simulink model "Kinematics_switch_sim"  (R2023b)
settings: Solver=ode15s  StartTime=0.0  StopTime=60  FixedStep=0.01  MaxStep=0.1  RelTol=1e-5
values from neighbouring files (symbols this model uses):
  a = 6.851221970532768e3    (= 6851.22197053)    [Kinematics_switch.m]
  A_313 = ( R_om * R_i * R_OM ).'    [Kinematics_switch.m]
  e = 0.001830122216180    (= 0.00183012221618)    [Kinematics_switch.m]
  I = diag([Ix Iy Iz])    [Kinematics_switch.m]
  I_inv = inv(I)    [Kinematics_switch.m]
  n = sqrt(mu / a^3)    [Kinematics_switch.m]
  s0 = [0; asin(0.4); pi/3]    [Kinematics_switch.m]
  theta0 = 3.109851878856139    (= 3.10985187886)    [Kinematics_switch.m]
  tol = 0.2    [Kinematics_switch.m]
  w0 = [0.5; -0.2; 1.0]    [Kinematics_switch.m]
libraries: simulink x2, matrix_library x1
settings Model: PauseTimes=53.05  Creator=turcu  LastModifiedBy=turcu

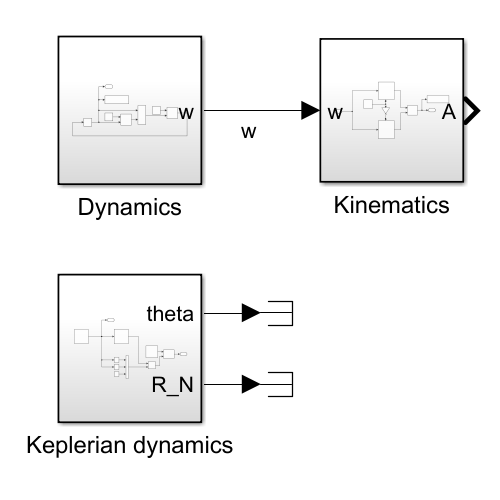
[thumbnail: Simulink's stored preview of the top-level diagram]
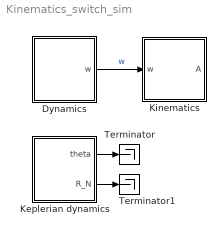
== system Kinematics_switch_sim ==
  Dynamics : Subsystem
  Keplerian dynamics : Subsystem
  Kinematics : Subsystem
  Terminator : Terminator
  Terminator1 : Terminator
  wires:
  Dynamics/1(w) -> Kinematics/1(w)  "w"
  Keplerian dynamics/1(theta) -> Terminator/1
  Keplerian dynamics/2(R_N) -> Terminator1/1

== system Kinematics_switch_sim/Dynamics ==
  Constant : Constant  Value=I
  Constant1 : Constant  Value=-I_inv
  Cross Product : matrix_library/Cross Product
  Integrator : Integrator  InitialCondition=w0
  Product : Product  Multiplication=Matrix(*)
  Product1 : Product  Multiplication=Matrix(*)
  To Workspace : ToWorkspace  VariableName=w  SaveFormat=Timeseries  SampleTime=-1
  w : Outport
  wires:
  Cross Product/1 -> Product1/2
  Constant/1 -> Product/1
  Integrator/1 -> Product/2, w/1, To Workspace/1, Cross Product/1  "w"
  Constant1/1 -> Product1/1
  Product/1 -> Cross Product/2
  Product1/1 -> Integrator/1  "wdot"

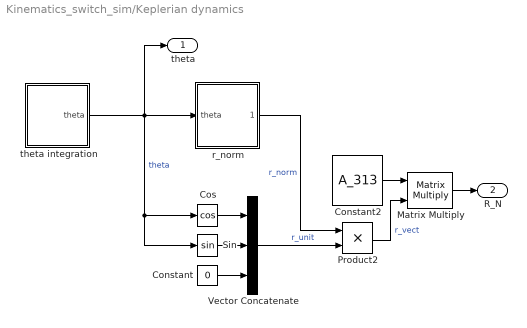
== system Kinematics_switch_sim/Keplerian dynamics ==
  Constant : Constant  Value=0
  Constant2 : Constant  Value=A_313
  Cos : Trigonometry  Operator=cos
  Matrix Multiply : Product  Multiplication=Matrix(*)
  Product2 : Product
  Sin : Trigonometry
  Vector Concatenate : Concatenate  NumInputs=3
  r_norm : Subsystem
  theta integration : Subsystem
  theta : Outport
  R_N : Outport  Port=2
  wires:
  Constant/1 -> Vector Concatenate/3
  Cos/1 -> Vector Concatenate/1
  r_norm/1(r_norm) -> Product2/1  "r_norm"
  Vector Concatenate/1 -> Product2/2  "r_unit"
  Sin/1 -> Vector Concatenate/2
  Constant2/1 -> Matrix Multiply/1
  Product2/1 -> Matrix Multiply/2  "r_vect"
  Matrix Multiply/1 -> R_N/1
  theta integration/1(theta) -> theta/1, Sin/1, Cos/1, r_norm/1(theta)  "theta"

== system Kinematics_switch_sim/Kinematics ==
  w : Inport
  Kinematics 312 : Subsystem
  Kinematics 313 : Subsystem
  Merge : Merge
  NOT : Logic  Operator=NOT  IconShape=distinctive  AllPortsSameDT=off  OutDataTypeStr=boolean
  System switcher : Subsystem
  To Workspace : ToWorkspace  VariableName=A  SaveFormat=Timeseries  SampleTime=-1
  A : Outport
  wires:
  NOT/1 -> Kinematics 313/Enable
  w/1 -> Kinematics 312/1(w), Kinematics 313/1(w)
  System switcher/1(flag) -> Kinematics 312/Enable, NOT/1
  Kinematics 313/1(A) -> Merge/2
  Merge/1 -> A/1, To Workspace/1  "A"
  Kinematics 312/1(A) -> Merge/1

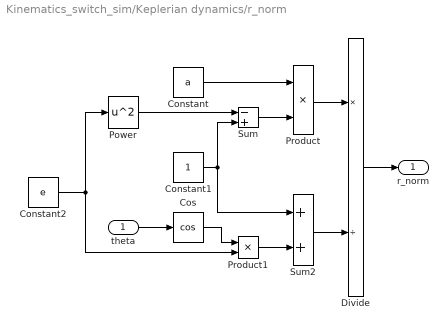
== system Kinematics_switch_sim/Keplerian dynamics/r_norm ==
  theta : Inport
  Constant : Constant  Value=a
  Constant1 : Constant
  Constant2 : Constant  Value=e
  Cos : Trigonometry  Operator=cos
  Divide : Product  Inputs=*/
  Power : Math  Operator=square
  Product : Product
  Product1 : Product
  Sum : Sum  Inputs=-+
  Sum2 : Sum
  r_norm : Outport
  wires:
  Constant2/1 -> Product1/2, Power/1
  Constant1/1 -> Sum/2, Sum2/1
  Sum/1 -> Product/2
  Constant/1 -> Product/1
  theta/1 -> Cos/1
  Cos/1 -> Product1/1
  Divide/1 -> r_norm/1
  Sum2/1 -> Divide/2
  Product/1 -> Divide/1
  Product1/1 -> Sum2/2
  Power/1 -> Sum/1

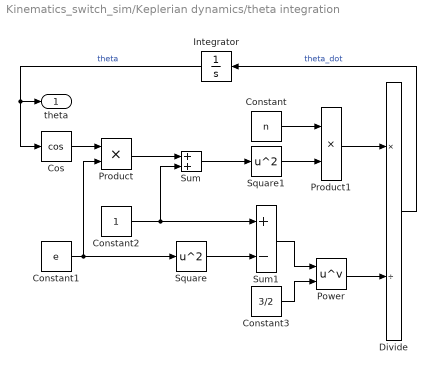
== system Kinematics_switch_sim/Keplerian dynamics/theta integration ==
  Constant : Constant  Value=n
  Constant1 : Constant  Value=e
  Constant2 : Constant
  Constant3 : Constant  Value=3/2
  Cos : Trigonometry  Operator=cos
  Divide : Product  Inputs=*/
  Integrator : Integrator  InitialCondition=theta0
  Power : Math  Operator=pow
  Product : Product
  Product1 : Product
  Square : Math  Operator=square
  Square1 : Math  Operator=square
  Sum : Sum
  Sum1 : Sum  Inputs=+-
  theta : Outport
  wires:
  Product1/1 -> Divide/1
  Power/1 -> Divide/2
  Sum1/1 -> Power/1
  Constant2/1 -> Sum/2, Sum1/1
  Square/1 -> Sum1/2
  Constant1/1 -> Product/2, Square/1
  Constant/1 -> Product1/1
  Sum/1 -> Square1/1
  Square1/1 -> Product1/2
  Cos/1 -> Product/1
  Divide/1 -> Integrator/1  "theta_dot"
  Integrator/1 -> theta/1, Cos/1  "theta"
  Constant3/1 -> Power/2
  Product/1 -> Sum/1

== system Kinematics_switch_sim/Kinematics/Kinematics 312 ==
  w : Inport
  Enable : EnablePort  StatesWhenEnabling=reset
  A - s_312 : Subsystem
  Euler angles : Subsystem
  IC : InitialCondition  Value=s0
  s_312 - A : Subsystem
  s_313 - A : Subsystem
  A : Outport
  wires:
  s_312 - A/1(A) -> A/1  "A"
  Euler angles/1(s) -> s_312 - A/1(s)  "s"
  w/1 -> Euler angles/1(w)
  IC/1 -> Euler angles/2(s0)
  A - s_312/1(s) -> IC/1
  s_313 - A/1(A) -> A - s_312/1(A)
  [s_313] -> s_313 - A/1(s)

== system Kinematics_switch_sim/Kinematics/Kinematics 313 ==
  w : Inport
  Enable : EnablePort  StatesWhenEnabling=reset
  A - s_313 : Subsystem
  Euler angles : Subsystem
  s_312 - A : Subsystem
  s_313 - A : Subsystem
  A : Outport
  wires:
  w/1 -> Euler angles/1(w)
  Euler angles/1(s) -> s_313 - A/1(s)
  s_313 - A/1(A) -> A/1
  A - s_313/1(s) -> Euler angles/2(s0)
  s_312 - A/1(A) -> A - s_313/1(A)
  [s_312] -> s_312 - A/1(s)

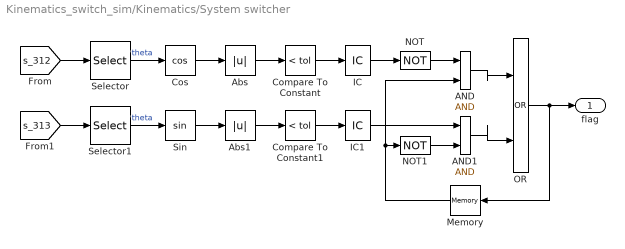
== system Kinematics_switch_sim/Kinematics/System switcher ==
  AND : Logic  IconShape=distinctive  AllPortsSameDT=off  OutDataTypeStr=boolean
  AND1 : Logic  IconShape=distinctive  AllPortsSameDT=off  OutDataTypeStr=boolean
  Abs : Abs  SaturateOnIntegerOverflow=off
  Abs1 : Abs  SaturateOnIntegerOverflow=off
  Compare To Constant : simulink/Logic and Bit Operations/Compare To Constant  relop=<  const=tol  OutDataTypeStr=boolean
  Compare To Constant1 : simulink/Logic and Bit Operations/Compare To Constant  relop=<  const=tol  OutDataTypeStr=boolean
  Cos : Trigonometry  Operator=cos
  IC : InitialCondition  Value=0
  IC1 : InitialCondition  Value=0
  Memory : Memory  InitialCondition=1
  NOT : Logic  Operator=NOT  IconShape=distinctive  AllPortsSameDT=off  OutDataTypeStr=boolean
  NOT1 : Logic  Operator=NOT  IconShape=distinctive  AllPortsSameDT=off  OutDataTypeStr=boolean
  OR : Logic  Operator=OR  IconShape=distinctive  AllPortsSameDT=off  OutDataTypeStr=boolean
  Selector : Selector  InputPortWidth=3  IndexOptions=Index vector (dialog)  Indices=2  OutputSizes=1
  Selector1 : Selector  InputPortWidth=3  IndexOptions=Index vector (dialog)  Indices=2  OutputSizes=1
  Sin : Trigonometry
  flag : Outport
  wires:
  Cos/1 -> Abs/1
  [s_312] -> Selector/1
  Compare To Constant/1 -> IC/1
  Selector1/1 -> Sin/1  "theta"
  Abs/1 -> Compare To Constant/1
  Compare To Constant1/1 -> IC1/1
  Selector/1 -> Cos/1  "theta"
  Abs1/1 -> Compare To Constant1/1
  Sin/1 -> Abs1/1
  [s_313] -> Selector1/1
  IC/1 -> NOT/1
  NOT/1 -> AND/1
  AND/1 -> OR/1
  NOT1/1 -> AND1/2
  IC1/1 -> AND1/1
  AND1/1 -> OR/2
  OR/1 -> Memory/1, flag/1
  Memory/1 -> AND/2, NOT1/1

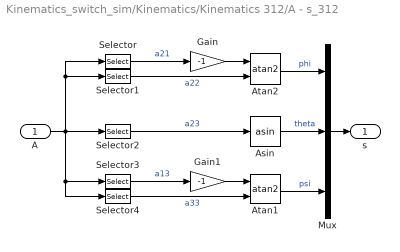
== system Kinematics_switch_sim/Kinematics/Kinematics 312/A - s_312 ==
  A : Inport
  Asin : Trigonometry  Operator=asin
  Atan1 : Trigonometry  Operator=atan2
  Atan2 : Trigonometry  Operator=atan2
  Gain : Gain  Gain=-1
  Gain1 : Gain  Gain=-1
  Mux : Mux  Inputs=3
  Selector : Selector  NumberOfDimensions=2  InputPortWidth=3  IndexOptions=Index vector (dialog),Index vector (dialog)  Indices=2,1  OutputSizes=1,1
  Selector1 : Selector  NumberOfDimensions=2  InputPortWidth=3  IndexOptions=Index vector (dialog),Index vector (dialog)  Indices=2,2  OutputSizes=1,1
  Selector2 : Selector  NumberOfDimensions=2  InputPortWidth=3  IndexOptions=Index vector (dialog),Index vector (dialog)  Indices=2,3  OutputSizes=1,1
  Selector3 : Selector  NumberOfDimensions=2  InputPortWidth=3  IndexOptions=Index vector (dialog),Index vector (dialog)  Indices=1,3  OutputSizes=1,1
  Selector4 : Selector  NumberOfDimensions=2  InputPortWidth=3  IndexOptions=Index vector (dialog),Index vector (dialog)  Indices=3,3  OutputSizes=1,1
  s : Outport
  wires:
  Mux/1 -> s/1
  Selector4/1 -> Atan1/2  "a33"
  Atan1/1 -> Mux/3  "psi"
  Atan2/1 -> Mux/1  "phi"
  A/1 -> Selector2/1, Selector1/1, Selector/1, Selector3/1, Selector4/1
  Selector2/1 -> Asin/1  "a23"
  Selector3/1 -> Gain1/1  "a13"
  Selector1/1 -> Atan2/2  "a22"
  Selector/1 -> Gain/1  "a21"
  Asin/1 -> Mux/2  "theta"
  Gain/1 -> Atan2/1
  Gain1/1 -> Atan1/1

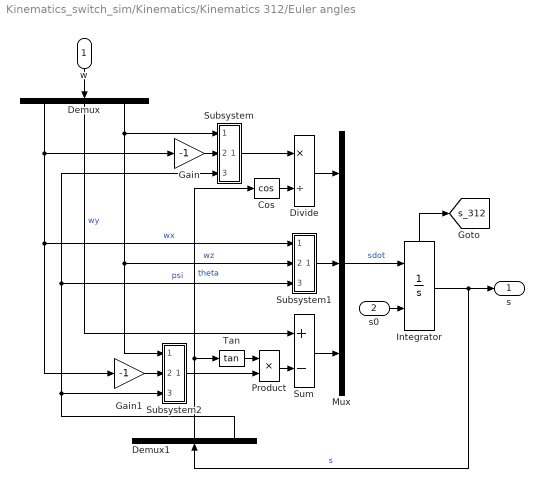
== system Kinematics_switch_sim/Kinematics/Kinematics 312/Euler angles ==
  w : Inport
  s0 : Inport  Port=2
  Cos : Trigonometry  Operator=cos
  Demux : Demux  Outputs=3
  Demux1 : Demux  Outputs=3
  Divide : Product  Inputs=*/
  Gain : Gain  Gain=-1
  Gain1 : Gain  Gain=-1
  Integrator : Integrator  InitialConditionSource=external  InitialCondition=s0  WrapState=on  WrappedStateUpperValue=2*pi  WrappedStateLowerValue=0  ShowStatePort=on
  Mux : Mux  Inputs=3
  Product : Product
  Subsystem : Subsystem
  Subsystem1 : Subsystem
  Subsystem2 : Subsystem
  Sum : Sum  Inputs=+-
  Tan : Trigonometry  Operator=tan
  s : Outport
  tag scope: s_312=global
  wires:
  w/1 -> Demux/1
  Integrator/1 -> Demux1/1, s/1  "s"
  Demux/3 -> Subsystem2/1(In1), Subsystem1/2(In2), Subsystem/1(In1)  "wz"
  Gain/1 -> Subsystem/2(In2)
  Demux/1 -> Gain1/1, Subsystem1/1(In1), Gain/1  "wx"
  Demux1/3 -> Subsystem2/3(In3), Subsystem1/3(In3), Subsystem/3(In3)  "psi"
  Subsystem/1(Out1) -> Divide/1
  Cos/1 -> Divide/2
  Demux1/2 -> Cos/1, Tan/1  "theta"
  Divide/1 -> Mux/1
  Subsystem1/1(Out1) -> Mux/2
  Gain1/1 -> Subsystem2/2(In2)
  Tan/1 -> Product/1
  Subsystem2/1(Out1) -> Product/2
  Product/1 -> Sum/2
  Demux/2 -> Sum/1  "wy"
  Sum/1 -> Mux/3
  Mux/1 -> Integrator/1  "sdot"
  s0/1 -> Integrator/2
  Integrator/State -> [s_312]

== system Kinematics_switch_sim/Kinematics/Kinematics 312/s_312 - A ==
  s : Inport
  Demux : Demux  Outputs=3
  Product : Product  Inputs=3  Multiplication=Matrix(*)
  R1 : Subsystem
  R2 : Subsystem
  R3 : Subsystem
  A : Outport
  wires:
  s/1 -> Demux/1  "s"
  R1/1(R1) -> Product/2
  R3/1(R3) -> Product/3
  R2/1(R2) -> Product/1
  Product/1 -> A/1
  Demux/2 -> R1/1(x)  "theta"
  Demux/1 -> R3/1(x)  "phi"
  Demux/3 -> R2/1(x)  "psi"

== system Kinematics_switch_sim/Kinematics/Kinematics 312/s_313 - A ==
  s : Inport
  Demux : Demux  Outputs=3
  Product : Product  Inputs=3  Multiplication=Matrix(*)
  R1 : Subsystem
  R3_1 : Subsystem
  R3_2 : Subsystem
  A : Outport
  wires:
  Demux/3 -> R3_2/1(x)  "psi"
  Demux/1 -> R3_1/1(x)  "phi"
  Demux/2 -> R1/1(x)  "theta"
  Product/1 -> A/1
  R1/1(R1) -> Product/2
  s/1 -> Demux/1  "s"
  R3_1/1(R3) -> Product/3
  R3_2/1(R3) -> Product/1

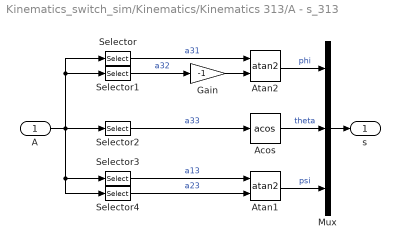
== system Kinematics_switch_sim/Kinematics/Kinematics 313/A - s_313 ==
  A : Inport
  Acos : Trigonometry  Operator=acos
  Atan1 : Trigonometry  Operator=atan2
  Atan2 : Trigonometry  Operator=atan2
  Gain : Gain  Gain=-1
  Mux : Mux  Inputs=3
  Selector : Selector  NumberOfDimensions=2  InputPortWidth=3  IndexOptions=Index vector (dialog),Index vector (dialog)  Indices=3,1  OutputSizes=1,1
  Selector1 : Selector  NumberOfDimensions=2  InputPortWidth=3  IndexOptions=Index vector (dialog),Index vector (dialog)  Indices=3,2  OutputSizes=1,1
  Selector2 : Selector  NumberOfDimensions=2  InputPortWidth=3  IndexOptions=Index vector (dialog),Index vector (dialog)  Indices=3,3  OutputSizes=1,1
  Selector3 : Selector  NumberOfDimensions=2  InputPortWidth=3  IndexOptions=Index vector (dialog),Index vector (dialog)  Indices=1,3  OutputSizes=1,1
  Selector4 : Selector  NumberOfDimensions=2  InputPortWidth=3  IndexOptions=Index vector (dialog),Index vector (dialog)  Indices=2,3  OutputSizes=1,1
  s : Outport
  wires:
  Acos/1 -> Mux/2  "theta"
  Selector/1 -> Atan2/1  "a31"
  Selector1/1 -> Gain/1  "a32"
  Selector3/1 -> Atan1/1  "a13"
  Selector2/1 -> Acos/1  "a33"
  A/1 -> Selector4/1, Selector3/1, Selector/1, Selector1/1, Selector2/1
  Atan2/1 -> Mux/1  "phi"
  Atan1/1 -> Mux/3  "psi"
  Gain/1 -> Atan2/2
  Selector4/1 -> Atan1/2  "a23"
  Mux/1 -> s/1

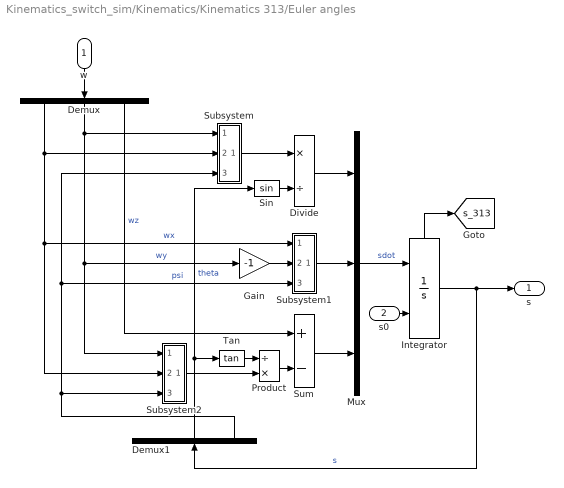
== system Kinematics_switch_sim/Kinematics/Kinematics 313/Euler angles ==
  w : Inport
  s0 : Inport  Port=2
  Demux : Demux  Outputs=3
  Demux1 : Demux  Outputs=3
  Divide : Product  Inputs=*/
  Gain : Gain  Gain=-1
  Integrator : Integrator  InitialConditionSource=external  InitialCondition=s0  WrapState=on  WrappedStateUpperValue=2*pi  WrappedStateLowerValue=0  ShowStatePort=on
  Mux : Mux  Inputs=3
  Product : Product  Inputs=/*
  Sin : Trigonometry
  Subsystem : Subsystem
  Subsystem1 : Subsystem
  Subsystem2 : Subsystem
  Sum : Sum  Inputs=+-
  Tan : Trigonometry  Operator=tan
  s : Outport
  tag scope: s_313=global
  wires:
  Mux/1 -> Integrator/1  "sdot"
  Sum/1 -> Mux/3
  Demux/2 -> Subsystem/1(In1), Subsystem2/1(In1), Gain/1  "wy"
  Product/1 -> Sum/2
  Subsystem2/1(Out1) -> Product/2
  Tan/1 -> Product/1
  Subsystem1/1(Out1) -> Mux/2
  Divide/1 -> Mux/1
  Demux1/2 -> Sin/1, Tan/1  "theta"
  Subsystem/1(Out1) -> Divide/1
  Demux1/3 -> Subsystem/3(In3), Subsystem1/3(In3), Subsystem2/3(In3)  "psi"
  Demux/1 -> Subsystem2/2(In2), Subsystem1/1(In1), Subsystem/2(In2)  "wx"
  Demux/3 -> Sum/1  "wz"
  Integrator/1 -> Demux1/1, s/1  "s"
  w/1 -> Demux/1
  Sin/1 -> Divide/2
  Gain/1 -> Subsystem1/2(In2)
  s0/1 -> Integrator/2
  Integrator/State -> [s_313]

== system Kinematics_switch_sim/Kinematics/Kinematics 313/s_312 - A ==
  s : Inport
  Demux : Demux  Outputs=3
  Product : Product  Inputs=3  Multiplication=Matrix(*)
  R1 : Subsystem
  R2 : Subsystem
  R3 : Subsystem
  A : Outport
  wires:
  s/1 -> Demux/1  "s"
  R1/1(R1) -> Product/2
  R3/1(R3) -> Product/3
  R2/1(R2) -> Product/1
  Product/1 -> A/1
  Demux/2 -> R1/1(x)  "theta"
  Demux/1 -> R3/1(x)  "phi"
  Demux/3 -> R2/1(x)  "psi"

== system Kinematics_switch_sim/Kinematics/Kinematics 313/s_313 - A ==
  s : Inport
  Demux : Demux  Outputs=3
  Product : Product  Inputs=3  Multiplication=Matrix(*)
  R1 : Subsystem
  R3_1 : Subsystem
  R3_2 : Subsystem
  A : Outport
  wires:
  Demux/3 -> R3_2/1(x)  "psi"
  Demux/1 -> R3_1/1(x)  "phi"
  Demux/2 -> R1/1(x)  "theta"
  Product/1 -> A/1
  R1/1(R1) -> Product/2
  s/1 -> Demux/1  "s"
  R3_1/1(R3) -> Product/3
  R3_2/1(R3) -> Product/1

== system Kinematics_switch_sim/Kinematics/Kinematics 312/Euler angles/Subsystem ==
  In1 : Inport
  In2 : Inport  Port=2
  In3 : Inport  Port=3
  Cos : Trigonometry  Operator=cos
  Product : Product
  Product1 : Product
  Sin : Trigonometry
  Sum : Sum
  Out1 : Outport
  wires:
  In3/1 -> Sin/1, Cos/1
  In1/1 -> Product/1
  Cos/1 -> Product/2
  Sin/1 -> Product1/1
  In2/1 -> Product1/2
  Product/1 -> Sum/1
  Product1/1 -> Sum/2
  Sum/1 -> Out1/1

== system Kinematics_switch_sim/Kinematics/Kinematics 312/Euler angles/Subsystem1 ==
  In1 : Inport
  In2 : Inport  Port=2
  In3 : Inport  Port=3
  Cos : Trigonometry  Operator=cos
  Product : Product
  Product1 : Product
  Sin : Trigonometry
  Sum : Sum
  Out1 : Outport
  wires:
  Sum/1 -> Out1/1
  Product1/1 -> Sum/2
  Product/1 -> Sum/1
  In2/1 -> Product1/2
  Sin/1 -> Product1/1
  Cos/1 -> Product/2
  In1/1 -> Product/1
  In3/1 -> Cos/1, Sin/1

== system Kinematics_switch_sim/Kinematics/Kinematics 312/Euler angles/Subsystem2 ==
  In1 : Inport
  In2 : Inport  Port=2
  In3 : Inport  Port=3
  Cos : Trigonometry  Operator=cos
  Product : Product
  Product1 : Product
  Sin : Trigonometry
  Sum : Sum
  Out1 : Outport
  wires:
  In3/1 -> Sin/1, Cos/1
  In1/1 -> Product/1
  Cos/1 -> Product/2
  Sin/1 -> Product1/1
  In2/1 -> Product1/2
  Product/1 -> Sum/1
  Product1/1 -> Sum/2
  Sum/1 -> Out1/1

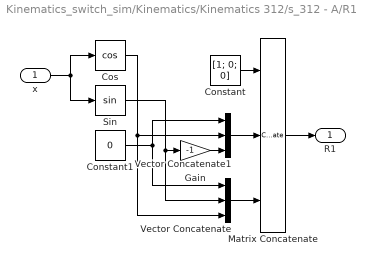
== system Kinematics_switch_sim/Kinematics/Kinematics 312/s_312 - A/R1 ==
  x : Inport
  Constant : Constant  Value=[1; 0; 0]
  Constant1 : Constant  Value=0
  Cos : Trigonometry  Operator=cos
  Gain : Gain  Gain=-1
  Matrix Concatenate : Concatenate  NumInputs=3  Mode=Multidimensional array  ConcatenateDimension=2
  Sin : Trigonometry
  Vector Concatenate : Concatenate  NumInputs=3
  Vector Concatenate1 : Concatenate  NumInputs=3
  R1 : Outport
  wires:
  Matrix Concatenate/1 -> R1/1
  x/1 -> Cos/1, Sin/1
  Vector Concatenate1/1 -> Matrix Concatenate/2
  Constant/1 -> Matrix Concatenate/1
  Vector Concatenate/1 -> Matrix Concatenate/3
  Constant1/1 -> Vector Concatenate/1, Vector Concatenate1/1
  Cos/1 -> Vector Concatenate/3, Vector Concatenate1/2
  Gain/1 -> Vector Concatenate1/3
  Sin/1 -> Vector Concatenate/2, Gain/1

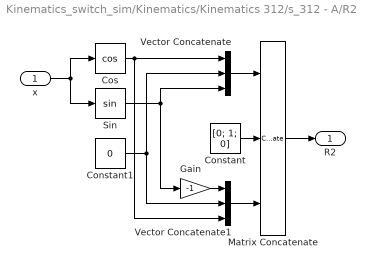
== system Kinematics_switch_sim/Kinematics/Kinematics 312/s_312 - A/R2 ==
  x : Inport
  Constant : Constant  Value=[0; 1; 0]
  Constant1 : Constant  Value=0
  Cos : Trigonometry  Operator=cos
  Gain : Gain  Gain=-1
  Matrix Concatenate : Concatenate  NumInputs=3  Mode=Multidimensional array  ConcatenateDimension=2
  Sin : Trigonometry
  Vector Concatenate : Concatenate  NumInputs=3
  Vector Concatenate1 : Concatenate  NumInputs=3
  R2 : Outport
  wires:
  Vector Concatenate/1 -> Matrix Concatenate/1
  x/1 -> Sin/1, Cos/1
  Matrix Concatenate/1 -> R2/1
  Constant/1 -> Matrix Concatenate/2
  Vector Concatenate1/1 -> Matrix Concatenate/3
  Constant1/1 -> Vector Concatenate/2, Vector Concatenate1/2
  Cos/1 -> Vector Concatenate1/3, Vector Concatenate/1
  Sin/1 -> Gain/1, Vector Concatenate/3
  Gain/1 -> Vector Concatenate1/1

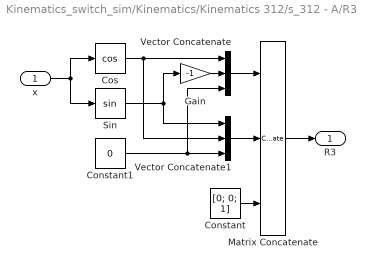
== system Kinematics_switch_sim/Kinematics/Kinematics 312/s_312 - A/R3 ==
  x : Inport
  Constant : Constant  Value=[0; 0; 1]
  Constant1 : Constant  Value=0
  Cos : Trigonometry  Operator=cos
  Gain : Gain  Gain=-1
  Matrix Concatenate : Concatenate  NumInputs=3  Mode=Multidimensional array  ConcatenateDimension=2
  Sin : Trigonometry
  Vector Concatenate : Concatenate  NumInputs=3
  Vector Concatenate1 : Concatenate  NumInputs=3
  R3 : Outport
  wires:
  Vector Concatenate/1 -> Matrix Concatenate/1
  Sin/1 -> Vector Concatenate1/1, Gain/1
  Cos/1 -> Vector Concatenate1/2, Vector Concatenate/1
  Constant/1 -> Matrix Concatenate/3
  Gain/1 -> Vector Concatenate/2
  Vector Concatenate1/1 -> Matrix Concatenate/2
  x/1 -> Sin/1, Cos/1
  Constant1/1 -> Vector Concatenate/3, Vector Concatenate1/3
  Matrix Concatenate/1 -> R3/1

== system Kinematics_switch_sim/Kinematics/Kinematics 312/s_313 - A/R1 ==
  x : Inport
  Constant : Constant  Value=[1; 0; 0]
  Constant1 : Constant  Value=0
  Cos : Trigonometry  Operator=cos
  Gain : Gain  Gain=-1
  Matrix Concatenate : Concatenate  NumInputs=3  Mode=Multidimensional array  ConcatenateDimension=2
  Sin : Trigonometry
  Vector Concatenate : Concatenate  NumInputs=3
  Vector Concatenate1 : Concatenate  NumInputs=3
  R1 : Outport
  wires:
  Sin/1 -> Gain/1, Vector Concatenate/2
  Gain/1 -> Vector Concatenate1/3
  Cos/1 -> Vector Concatenate1/2, Vector Concatenate/3
  Constant1/1 -> Vector Concatenate1/1, Vector Concatenate/1
  Vector Concatenate/1 -> Matrix Concatenate/3
  Constant/1 -> Matrix Concatenate/1
  Vector Concatenate1/1 -> Matrix Concatenate/2
  x/1 -> Sin/1, Cos/1
  Matrix Concatenate/1 -> R1/1

== system Kinematics_switch_sim/Kinematics/Kinematics 312/s_313 - A/R3_1 ==
  x : Inport
  Constant : Constant  Value=[0; 0; 1]
  Constant1 : Constant  Value=0
  Cos : Trigonometry  Operator=cos
  Gain : Gain  Gain=-1
  Matrix Concatenate : Concatenate  NumInputs=3  Mode=Multidimensional array  ConcatenateDimension=2
  Sin : Trigonometry
  Vector Concatenate : Concatenate  NumInputs=3
  Vector Concatenate1 : Concatenate  NumInputs=3
  R3 : Outport
  wires:
  Matrix Concatenate/1 -> R3/1
  Constant1/1 -> Vector Concatenate1/3, Vector Concatenate/3
  x/1 -> Cos/1, Sin/1
  Vector Concatenate1/1 -> Matrix Concatenate/2
  Gain/1 -> Vector Concatenate/2
  Constant/1 -> Matrix Concatenate/3
  Cos/1 -> Vector Concatenate/1, Vector Concatenate1/2
  Sin/1 -> Gain/1, Vector Concatenate1/1
  Vector Concatenate/1 -> Matrix Concatenate/1

== system Kinematics_switch_sim/Kinematics/Kinematics 312/s_313 - A/R3_2 ==
  x : Inport
  Constant : Constant  Value=[0; 0; 1]
  Constant1 : Constant  Value=0
  Cos : Trigonometry  Operator=cos
  Gain : Gain  Gain=-1
  Matrix Concatenate : Concatenate  NumInputs=3  Mode=Multidimensional array  ConcatenateDimension=2
  Sin : Trigonometry
  Vector Concatenate : Concatenate  NumInputs=3
  Vector Concatenate1 : Concatenate  NumInputs=3
  R3 : Outport
  wires:
  Vector Concatenate/1 -> Matrix Concatenate/1
  Sin/1 -> Vector Concatenate1/1, Gain/1
  Cos/1 -> Vector Concatenate1/2, Vector Concatenate/1
  Constant/1 -> Matrix Concatenate/3
  Gain/1 -> Vector Concatenate/2
  Vector Concatenate1/1 -> Matrix Concatenate/2
  x/1 -> Sin/1, Cos/1
  Constant1/1 -> Vector Concatenate/3, Vector Concatenate1/3
  Matrix Concatenate/1 -> R3/1

== system Kinematics_switch_sim/Kinematics/Kinematics 313/Euler angles/Subsystem ==
  In1 : Inport
  In2 : Inport  Port=2
  In3 : Inport  Port=3
  Cos : Trigonometry  Operator=cos
  Product : Product
  Product1 : Product
  Sin : Trigonometry
  Sum : Sum
  Out1 : Outport
  wires:
  Sum/1 -> Out1/1
  Product1/1 -> Sum/2
  Product/1 -> Sum/1
  In2/1 -> Product1/2
  Sin/1 -> Product1/1
  Cos/1 -> Product/2
  In1/1 -> Product/1
  In3/1 -> Cos/1, Sin/1

== system Kinematics_switch_sim/Kinematics/Kinematics 313/Euler angles/Subsystem1 ==
  In1 : Inport
  In2 : Inport  Port=2
  In3 : Inport  Port=3
  Cos : Trigonometry  Operator=cos
  Product : Product
  Product1 : Product
  Sin : Trigonometry
  Sum : Sum
  Out1 : Outport
  wires:
  In3/1 -> Sin/1, Cos/1
  In1/1 -> Product/1
  Cos/1 -> Product/2
  Sin/1 -> Product1/1
  In2/1 -> Product1/2
  Product/1 -> Sum/1
  Product1/1 -> Sum/2
  Sum/1 -> Out1/1

== system Kinematics_switch_sim/Kinematics/Kinematics 313/Euler angles/Subsystem2 ==
  In1 : Inport
  In2 : Inport  Port=2
  In3 : Inport  Port=3
  Cos : Trigonometry  Operator=cos
  Product : Product
  Product1 : Product
  Sin : Trigonometry
  Sum : Sum
  Out1 : Outport
  wires:
  Sum/1 -> Out1/1
  Product1/1 -> Sum/2
  Product/1 -> Sum/1
  In2/1 -> Product1/2
  Sin/1 -> Product1/1
  Cos/1 -> Product/2
  In1/1 -> Product/1
  In3/1 -> Cos/1, Sin/1

== system Kinematics_switch_sim/Kinematics/Kinematics 313/s_312 - A/R1 ==
  x : Inport
  Constant : Constant  Value=[1; 0; 0]
  Constant1 : Constant  Value=0
  Cos : Trigonometry  Operator=cos
  Gain : Gain  Gain=-1
  Matrix Concatenate : Concatenate  NumInputs=3  Mode=Multidimensional array  ConcatenateDimension=2
  Sin : Trigonometry
  Vector Concatenate : Concatenate  NumInputs=3
  Vector Concatenate1 : Concatenate  NumInputs=3
  R1 : Outport
  wires:
  Matrix Concatenate/1 -> R1/1
  x/1 -> Cos/1, Sin/1
  Vector Concatenate1/1 -> Matrix Concatenate/2
  Constant/1 -> Matrix Concatenate/1
  Vector Concatenate/1 -> Matrix Concatenate/3
  Constant1/1 -> Vector Concatenate/1, Vector Concatenate1/1
  Cos/1 -> Vector Concatenate/3, Vector Concatenate1/2
  Gain/1 -> Vector Concatenate1/3
  Sin/1 -> Vector Concatenate/2, Gain/1

== system Kinematics_switch_sim/Kinematics/Kinematics 313/s_312 - A/R2 ==
  x : Inport
  Constant : Constant  Value=[0; 1; 0]
  Constant1 : Constant  Value=0
  Cos : Trigonometry  Operator=cos
  Gain : Gain  Gain=-1
  Matrix Concatenate : Concatenate  NumInputs=3  Mode=Multidimensional array  ConcatenateDimension=2
  Sin : Trigonometry
  Vector Concatenate : Concatenate  NumInputs=3
  Vector Concatenate1 : Concatenate  NumInputs=3
  R2 : Outport
  wires:
  Vector Concatenate/1 -> Matrix Concatenate/1
  x/1 -> Sin/1, Cos/1
  Matrix Concatenate/1 -> R2/1
  Constant/1 -> Matrix Concatenate/2
  Vector Concatenate1/1 -> Matrix Concatenate/3
  Constant1/1 -> Vector Concatenate/2, Vector Concatenate1/2
  Cos/1 -> Vector Concatenate1/3, Vector Concatenate/1
  Sin/1 -> Gain/1, Vector Concatenate/3
  Gain/1 -> Vector Concatenate1/1

== system Kinematics_switch_sim/Kinematics/Kinematics 313/s_312 - A/R3 ==
  x : Inport
  Constant : Constant  Value=[0; 0; 1]
  Constant1 : Constant  Value=0
  Cos : Trigonometry  Operator=cos
  Gain : Gain  Gain=-1
  Matrix Concatenate : Concatenate  NumInputs=3  Mode=Multidimensional array  ConcatenateDimension=2
  Sin : Trigonometry
  Vector Concatenate : Concatenate  NumInputs=3
  Vector Concatenate1 : Concatenate  NumInputs=3
  R3 : Outport
  wires:
  Vector Concatenate/1 -> Matrix Concatenate/1
  Sin/1 -> Vector Concatenate1/1, Gain/1
  Cos/1 -> Vector Concatenate1/2, Vector Concatenate/1
  Constant/1 -> Matrix Concatenate/3
  Gain/1 -> Vector Concatenate/2
  Vector Concatenate1/1 -> Matrix Concatenate/2
  x/1 -> Sin/1, Cos/1
  Constant1/1 -> Vector Concatenate/3, Vector Concatenate1/3
  Matrix Concatenate/1 -> R3/1

== system Kinematics_switch_sim/Kinematics/Kinematics 313/s_313 - A/R1 ==
  x : Inport
  Constant : Constant  Value=[1; 0; 0]
  Constant1 : Constant  Value=0
  Cos : Trigonometry  Operator=cos
  Gain : Gain  Gain=-1
  Matrix Concatenate : Concatenate  NumInputs=3  Mode=Multidimensional array  ConcatenateDimension=2
  Sin : Trigonometry
  Vector Concatenate : Concatenate  NumInputs=3
  Vector Concatenate1 : Concatenate  NumInputs=3
  R1 : Outport
  wires:
  Sin/1 -> Gain/1, Vector Concatenate/2
  Gain/1 -> Vector Concatenate1/3
  Cos/1 -> Vector Concatenate1/2, Vector Concatenate/3
  Constant1/1 -> Vector Concatenate1/1, Vector Concatenate/1
  Vector Concatenate/1 -> Matrix Concatenate/3
  Constant/1 -> Matrix Concatenate/1
  Vector Concatenate1/1 -> Matrix Concatenate/2
  x/1 -> Sin/1, Cos/1
  Matrix Concatenate/1 -> R1/1

== system Kinematics_switch_sim/Kinematics/Kinematics 313/s_313 - A/R3_1 ==
  x : Inport
  Constant : Constant  Value=[0; 0; 1]
  Constant1 : Constant  Value=0
  Cos : Trigonometry  Operator=cos
  Gain : Gain  Gain=-1
  Matrix Concatenate : Concatenate  NumInputs=3  Mode=Multidimensional array  ConcatenateDimension=2
  Sin : Trigonometry
  Vector Concatenate : Concatenate  NumInputs=3
  Vector Concatenate1 : Concatenate  NumInputs=3
  R3 : Outport
  wires:
  Matrix Concatenate/1 -> R3/1
  Constant1/1 -> Vector Concatenate1/3, Vector Concatenate/3
  x/1 -> Cos/1, Sin/1
  Vector Concatenate1/1 -> Matrix Concatenate/2
  Gain/1 -> Vector Concatenate/2
  Constant/1 -> Matrix Concatenate/3
  Cos/1 -> Vector Concatenate/1, Vector Concatenate1/2
  Sin/1 -> Gain/1, Vector Concatenate1/1
  Vector Concatenate/1 -> Matrix Concatenate/1

== system Kinematics_switch_sim/Kinematics/Kinematics 313/s_313 - A/R3_2 ==
  x : Inport
  Constant : Constant  Value=[0; 0; 1]
  Constant1 : Constant  Value=0
  Cos : Trigonometry  Operator=cos
  Gain : Gain  Gain=-1
  Matrix Concatenate : Concatenate  NumInputs=3  Mode=Multidimensional array  ConcatenateDimension=2
  Sin : Trigonometry
  Vector Concatenate : Concatenate  NumInputs=3
  Vector Concatenate1 : Concatenate  NumInputs=3
  R3 : Outport
  wires:
  Vector Concatenate/1 -> Matrix Concatenate/1
  Sin/1 -> Vector Concatenate1/1, Gain/1
  Cos/1 -> Vector Concatenate1/2, Vector Concatenate/1
  Constant/1 -> Matrix Concatenate/3
  Gain/1 -> Vector Concatenate/2
  Vector Concatenate1/1 -> Matrix Concatenate/2
  x/1 -> Sin/1, Cos/1
  Constant1/1 -> Vector Concatenate/3, Vector Concatenate1/3
  Matrix Concatenate/1 -> R3/1
